simulink model "IEEE_34_node_2018a"  (R2018a)
settings: Solver=FixedStepDiscrete  StartTime=0.0  StopTime=0.01  RelTol=1e-3
InitFcn:
  | power_34NodeTestFeeder_init;
  | power_34NodeTestFeeder_loads_init;
  | %=============================
  | Vnom_ph_ph = 24900;
  | Vnom = 24900/sqrt(3);
  | Vnom1_ph_ph = 4160;
  | Vnom1 = 4160/sqrt(3);
  | Degrees_ph_ph_gen1 = 0;
  | Frequency = 60;
  | Apparent_power_gen1 = 2500e3;
  | SW1 = 0;
values from neighbouring files (symbols this model uses):
  Pa_802_806 = [1e-6 30 25]*1e3    [power_34NodeTestFeeder_loads_init.m]
  Pa_808_810 = 16e3    (= 16000)    [power_34NodeTestFeeder_loads_init.m]
  Pa_816_824 = [1e-6 5 1e-6]*1e3    [power_34NodeTestFeeder_loads_init.m]
  Pa_818_820 = 34e3    (= 34000)    [power_34NodeTestFeeder_loads_init.m]
  Pa_820_822 = 135e3    (= 135000)    [power_34NodeTestFeeder_loads_init.m]
  Pa_824_826 = 40e3    (= 40000)    [power_34NodeTestFeeder_loads_init.m]
  Pa_824_828 = [1e-6 1e-6 4]*1e3    [power_34NodeTestFeeder_loads_init.m]
  Pa_828_830 = [7 1e-6 1e-6]*1e3    [power_34NodeTestFeeder_loads_init.m]
  Pa_832_858 = [7 2 6]*1e3    [power_34NodeTestFeeder_loads_init.m]
  Pa_834_860 = [16 20 110]*1e3    [power_34NodeTestFeeder_loads_init.m]
  Pa_836_840 = [18 22 1e-6]*1e3    [power_34NodeTestFeeder_loads_init.m]
  Pa_842_844 = [9 1e-6 1e-6]*1e3    [power_34NodeTestFeeder_loads_init.m]
  Pa_844_846 = [1e-6 25 20]*1e3    [power_34NodeTestFeeder_loads_init.m]
  Pa_846_848 = [1e-6 23 1e-6]*1e3    [power_34NodeTestFeeder_loads_init.m]
  Pa_854_856 = 4e3    (= 4000)    [power_34NodeTestFeeder_loads_init.m]
  Pa_858_834 = [4 15 13]*1e3    [power_34NodeTestFeeder_loads_init.m]
  Pa_858_864 = 2e3    (= 2000)    [power_34NodeTestFeeder_loads_init.m]
  Pa_860_836 = [30 10 42]*1e3    [power_34NodeTestFeeder_loads_init.m]
  Pa_862_838 = 28e3    (= 28000)    [power_34NodeTestFeeder_loads_init.m]
  Pp_802_806 = [1e-6 15 14]*1e3    [power_34NodeTestFeeder_loads_init.m]
  Pp_808_810 = 8e3    (= 8000)    [power_34NodeTestFeeder_loads_init.m]
  Pp_816_824 = [1e-6 2 1e-6]*1e3    [power_34NodeTestFeeder_loads_init.m]
  Pp_818_820 = 17e3    (= 17000)    [power_34NodeTestFeeder_loads_init.m]
  Pp_820_822 = 70e3    (= 70000)    [power_34NodeTestFeeder_loads_init.m]
  Pp_824_826 = 20e3    (= 20000)    [power_34NodeTestFeeder_loads_init.m]
  Pp_824_828 = [1e-6 1e-6 2]*1e3    [power_34NodeTestFeeder_loads_init.m]
  Pp_828_830 = [3 1e-6 1e-6]*1e3    [power_34NodeTestFeeder_loads_init.m]
  Pp_832_858 = [3 1 3]*1e3    [power_34NodeTestFeeder_loads_init.m]
  Pp_834_860 = [8 10 55]*1e3    [power_34NodeTestFeeder_loads_init.m]
  Pp_836_840 = [9 11 1e-6]*1e3    [power_34NodeTestFeeder_loads_init.m]
  Pp_842_844 = [5 1e-6 1e-6]*1e3    [power_34NodeTestFeeder_loads_init.m]
  Pp_844_846 = [1e-6 12 11]*1e3    [power_34NodeTestFeeder_loads_init.m]
  Pp_846_848 = [1e-6 11 1e-6]*1e3    [power_34NodeTestFeeder_loads_init.m]
  Pp_854_856 = 2e3    (= 2000)    [power_34NodeTestFeeder_loads_init.m]
  Pp_858_834 = [2 8 7]*1e3    [power_34NodeTestFeeder_loads_init.m]
  Pp_858_864 = 1e3    (= 1000)    [power_34NodeTestFeeder_loads_init.m]
  Pp_860_836 = [15 6 22]*1e3    [power_34NodeTestFeeder_loads_init.m]
  Pp_862_838 = 14e3    (= 14000)    [power_34NodeTestFeeder_loads_init.m]
  V_802_806 = [1.047 1.048 1.048]    [power_34NodeTestFeeder_loads_init.m]
  V_808_810 = 1.014    [power_34NodeTestFeeder_loads_init.m]
  V_816_824 = [1.017 1.025 1.02]*sqrt(3)    [power_34NodeTestFeeder_loads_init.m]
  V_818_820 = 1.016    [power_34NodeTestFeeder_loads_init.m]
  V_820_822 = 0.993    [power_34NodeTestFeeder_loads_init.m]
  V_824_826 = 1.008    [power_34NodeTestFeeder_loads_init.m]
  V_824_828 = [1.008 1.016 1.012]    [power_34NodeTestFeeder_loads_init.m]
  V_828_830 = [1.007 1.015 1.011]    [power_34NodeTestFeeder_loads_init.m]
  V_830 = [0.989 0.998 0.994]*sqrt(3)    [power_34NodeTestFeeder_loads_init.m]
  V_832_858 = [1.036 1.035 1.036]*sqrt(3)    [power_34NodeTestFeeder_loads_init.m]
  V_834_860 = [1.031 1.029 1.031]*sqrt(3)    [power_34NodeTestFeeder_loads_init.m]
  V_836_840 = [1.03 1.029 1.031]*sqrt(3)    [power_34NodeTestFeeder_loads_init.m]
  V_840 = [1.03 1.029 1.031]    [power_34NodeTestFeeder_loads_init.m]
  V_842_844 = [1.031 1.029 1.031]    [power_34NodeTestFeeder_loads_init.m]
  V_844 = [1.031 1.029 1.031]    [power_34NodeTestFeeder_loads_init.m]
  V_844_846 = [1.031 1.029 1.031]    [power_34NodeTestFeeder_loads_init.m]
  V_846_848 = [1.031 1.029 1.031]    [power_34NodeTestFeeder_loads_init.m]
  V_848 = [1.031 1.029 1.031]*sqrt(3)    [power_34NodeTestFeeder_loads_init.m]
  V_854_856 = 0.998    [power_34NodeTestFeeder_loads_init.m]
  V_858_834 = [1.034 1.032 1.034]*sqrt(3)    [power_34NodeTestFeeder_loads_init.m]
  V_860 = [1.03 1.029 1.031]    [power_34NodeTestFeeder_loads_init.m]
  V_860_836 = [1.03 1.029 1.031]*sqrt(3)    [power_34NodeTestFeeder_loads_init.m]
  V_862_838 = 1.029    [power_34NodeTestFeeder_loads_init.m]
  V_890 = [0.917 0.924 0.918]*sqrt(3)    [power_34NodeTestFeeder_loads_init.m]
undefined symbols (not defined in the file or in its folder): Angle, C_300, C_301, C_302, C_303, C_304, Degrees_ph, ft2km, L_300, L_301, L_302, L_303, L_304, Magnitude, ph, ph_gen1, R_300, R_301, R_302, R_303, R_304, Vnom_ph
libraries: powerlib x148
(part 2 of 2)

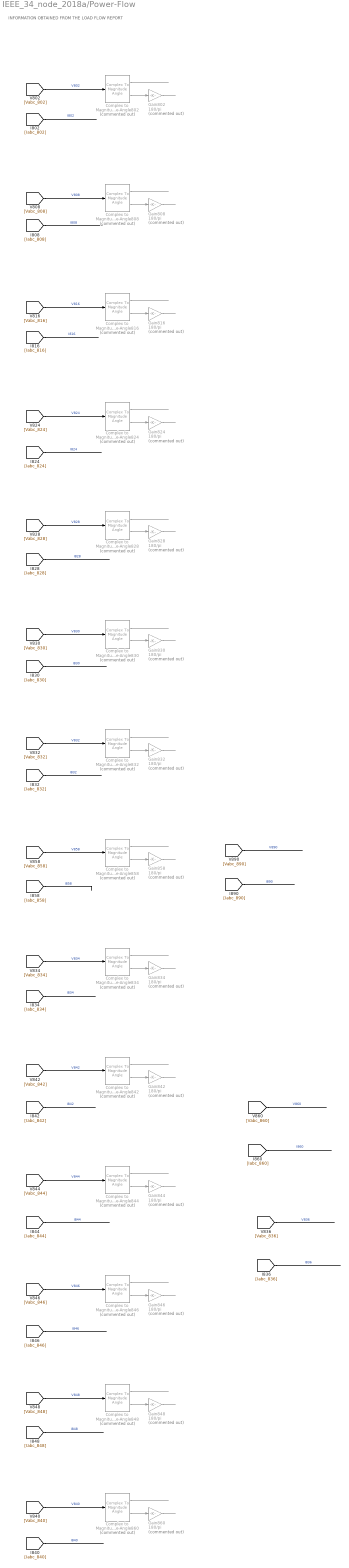
== system IEEE_34_node_2018a/Power-Flow ==
  note: INFORMATION OBTAINED FROM THE LOAD FLOW REPORT
  Complex to Magnitude-Angle{802,808,816,824,828,830,832,834,842,844,846,848,858,860} (14 alike) : ComplexToMagnitudeAngle  Commented=on
  Gain{802,808,816,824,828,830,832,834,842,844,846,848,858,860} (14 alike) : Gain  Commented=on  Gain=180/pi
  wires:
  [Vabc_808] -> Complex to Magnitude-Angle808/1  "V808"
  Complex to Magnitude-Angle808/2 -> Gain808/1
  Gain808/1 -> ?
  Complex to Magnitude-Angle808/1 -> ?
  Gain802/1 -> ?
  Complex to Magnitude-Angle802/2 -> Gain802/1
  [Vabc_802] -> Complex to Magnitude-Angle802/1  "V802"
  Complex to Magnitude-Angle802/1 -> ?
  Gain816/1 -> ?
  Complex to Magnitude-Angle816/2 -> Gain816/1
  [Vabc_816] -> Complex to Magnitude-Angle816/1  "V816"
  Complex to Magnitude-Angle816/1 -> ?
  [Vabc_824] -> Complex to Magnitude-Angle824/1  "V824"
  Complex to Magnitude-Angle824/2 -> Gain824/1
  Gain824/1 -> ?
  Complex to Magnitude-Angle824/1 -> ?
  Complex to Magnitude-Angle828/2 -> Gain828/1
  Complex to Magnitude-Angle828/1 -> ?
  [Vabc_828] -> Complex to Magnitude-Angle828/1  "V828"
  Gain828/1 -> ?
  Complex to Magnitude-Angle830/2 -> Gain830/1
  Complex to Magnitude-Angle830/1 -> ?
  [Vabc_830] -> Complex to Magnitude-Angle830/1  "V830"
  Gain830/1 -> ?
  Complex to Magnitude-Angle832/2 -> Gain832/1
  Complex to Magnitude-Angle832/1 -> ?
  [Vabc_832] -> Complex to Magnitude-Angle832/1  "V832"
  Gain832/1 -> ?
  Complex to Magnitude-Angle858/2 -> Gain858/1
  Complex to Magnitude-Angle858/1 -> ?
  [Vabc_858] -> Complex to Magnitude-Angle858/1  "V858"
  Gain858/1 -> ?
  Complex to Magnitude-Angle834/2 -> Gain834/1
  Complex to Magnitude-Angle834/1 -> ?
  [Vabc_834] -> Complex to Magnitude-Angle834/1  "V834"
  Gain834/1 -> ?
  Complex to Magnitude-Angle842/2 -> Gain842/1
  Complex to Magnitude-Angle842/1 -> ?
  [Vabc_842] -> Complex to Magnitude-Angle842/1  "V842"
  Gain842/1 -> ?
  Complex to Magnitude-Angle844/2 -> Gain844/1
  Complex to Magnitude-Angle844/1 -> ?
  [Vabc_844] -> Complex to Magnitude-Angle844/1  "V844"
  Gain844/1 -> ?
  Complex to Magnitude-Angle846/2 -> Gain846/1
  Complex to Magnitude-Angle846/1 -> ?
  [Vabc_846] -> Complex to Magnitude-Angle846/1  "V846"
  Gain846/1 -> ?
  Complex to Magnitude-Angle848/2 -> Gain848/1
  Complex to Magnitude-Angle848/1 -> ?
  [Vabc_848] -> Complex to Magnitude-Angle848/1  "V848"
  Gain848/1 -> ?
  Complex to Magnitude-Angle860/2 -> Gain860/1
  Complex to Magnitude-Angle860/1 -> ?
  [Vabc_840] -> Complex to Magnitude-Angle860/1  "V840"
  Gain860/1 -> ?
  [Iabc_802] -> ?  "I802"
  [Iabc_808] -> ?  "I808"
  [Iabc_816] -> ?  "I816"
  [Iabc_824] -> ?  "I824"
  [Iabc_828] -> ?  "I828"
  [Iabc_830] -> ?  "I830"
  [Iabc_832] -> ?  "I832"
  [Iabc_858] -> ?  "I858"
  [Iabc_834] -> ?  "I834"
  [Iabc_890] -> ?  "I890"
  [Vabc_890] -> ?  "V890"
  [Iabc_842] -> ?  "I842"
  [Iabc_844] -> ?  "I844"
  [Vabc_860] -> ?  "V860"
  [Iabc_860] -> ?  "I860"
  [Vabc_836] -> ?  "V836"
  [Iabc_836] -> ?  "I836"
  [Iabc_846] -> ?  "I846"
  [Iabc_848] -> ?  "I848"
  [Iabc_840] -> ?  "I840"
